simulink model "modelo"  (Simulink 8.3)
settings: Solver=ode45  StartTime=0.0  StopTime=Ts  RelTol=1e-3
values from neighbouring files (symbols this model uses):
  C1 = CC(j,1)    [Analsis.m]
  C2 = CC(j,2)    [Analsis.m]
  Cv = 1.6e-4    (= 0.00016)    [Analsis.m]
  D = 0.4    [Analsis.m]
  dt = 5    [Analsis.m]
  L = 0.6    [Analsis.m]
undefined symbols (not defined in the file or in its folder): U, Y
settings Model: Creator=Juan  LastModifiedBy=juand
settings OptimizationCC: ExpressionDepthLimit=2147483647
settings DebuggingCC: FcnCallInpInsideContextMsg=UseLocalSettings

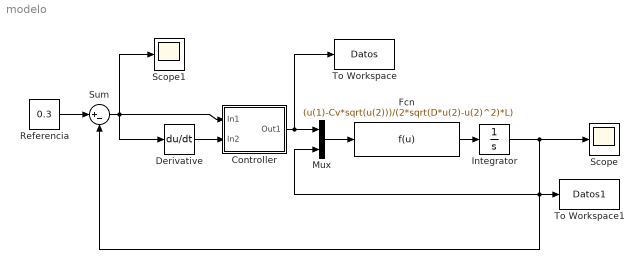
== system modelo ==
  Controller : Subsystem
  Derivative : Derivative
  Fcn : Fcn  Expr=(u(1)-Cv*sqrt(u(2)))/(2*sqrt(D*u(2)-u(2)^2)*L)  SampleTime=dt
  Integrator : Integrator  InitialCondition=0.01
  Mux : Mux  Inputs=2
  Referencia : Constant  Value=0.3
  Scope : Scope
      settings: YMin=0.01  YMax=0.17
  Scope1 : Scope
  Sum : Sum  Inputs=|+-
  To Workspace : ToWorkspace  VariableName=Datos  SaveFormat=Structure  SampleTime=-1
  To Workspace1 : ToWorkspace  VariableName=Datos1  SaveFormat=Structure  SampleTime=-1
  wires:
  Fcn/1 -> Integrator/1
  Integrator/1 -> Scope/1, Sum/2, Mux/2, To Workspace1/1
  Sum/1 -> Derivative/1, Scope1/1, Controller/1(In1)
  Referencia/1 -> Sum/1
  Mux/1 -> Fcn/1
  Derivative/1 -> Controller/2(In2)
  Controller/1(Out1) -> Mux/1, To Workspace/1

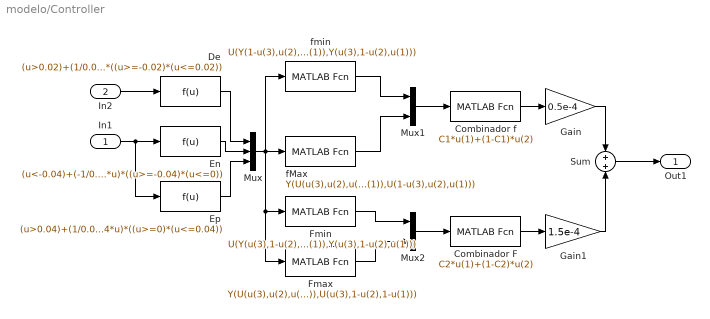
== system modelo/Controller ==
  In1 : Inport
  In2 : Inport  Port=2
  Combinador F : MATLABFcn  MATLABFcn=C2*u(1)+(1-C2)*u(2)
  Combinador f : MATLABFcn  MATLABFcn=C1*u(1)+(1-C1)*u(2)
  De : Fcn  Expr=(u>0.02)+(1/0.04*u+0.5)*((u>=-0.02)*(u<=0.02))
  En : Fcn  Expr=(u<-0.04)+(-1/0.04*u)*((u>=-0.04)*(u<=0))
  Ep : Fcn  Expr=(u>0.04)+(1/0.04*u)*((u>=0)*(u<=0.04))
  Fmax : MATLABFcn  MATLABFcn=Y(U(u(3),u(2),u(1)),U(u(3),u(2),1-u(1)),U(u(3),1-u(2),u(1)),U(u(3),1-u(2),1-u(1)))
  Fmin : MATLABFcn  MATLABFcn=U(Y(u(3),1-u(2),1-u(1)),Y(u(3),1-u(2),u(1)))
  Gain : Gain  Gain=0.5e-4
  Gain1 : Gain  Gain=1.5e-4
  Mux : Mux  Inputs=3
  Mux1 : Mux  Inputs=2
  Mux2 : Mux  Inputs=2
  Sum : Sum  Inputs=+|+
  fMax : MATLABFcn  MATLABFcn=Y(U(u(3),u(2),u(1)),U(u(3),u(2),1-u(1)),U(1-u(3),u(2),u(1)))
  fmin : MATLABFcn  MATLABFcn=U(Y(1-u(3),u(2),1-u(1)),Y(1-u(3),u(2),u(1)),Y(u(3),1-u(2),u(1)))
  Out1 : Outport
  wires:
  In1/1 -> Ep/1, En/1
  In2/1 -> De/1
  De/1 -> Mux/1
  En/1 -> Mux/2
  Ep/1 -> Mux/3
  Mux/1 -> fmin/1, fMax/1, Fmin/1, Fmax/1
  Mux1/1 -> Combinador f/1
  fmin/1 -> Mux1/1
  fMax/1 -> Mux1/2
  Mux2/1 -> Combinador F/1
  Fmin/1 -> Mux2/1
  Fmax/1 -> Mux2/2
  Combinador f/1 -> Gain/1
  Gain/1 -> Sum/1
  Combinador F/1 -> Gain1/1
  Gain1/1 -> Sum/2
  Sum/1 -> Out1/1
